simulink model "controlador_PID"  (R2018a)
settings: Solver=VariableStepAuto  StartTime=0.0  StopTime=10.0  RelTol=1e-3
values from neighbouring files (symbols this model uses):
  b_a = J_eq * n * w_pos    (= 0.0113019895361)    [proyecto_global_integrador.m]
  k_sa = J_eq * n * w_pos^2    (= 9.04159162887)    [proyecto_global_integrador.m]
  k_sia = J_eq * w_pos^3    (= 2893.30932124)    [proyecto_global_integrador.m]
settings Model: Creator=gabrielq  LastModifiedBy=gabrielq

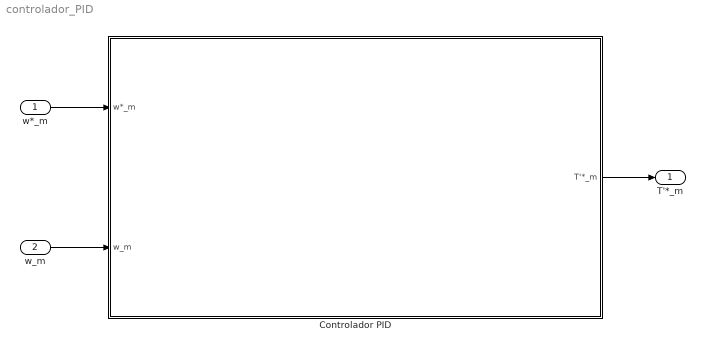
== system controlador_PID ==
  w*_m : Inport
  w_m : Inport  Port=2
  Controlador PID : Subsystem
  T'*_m : Outport
  wires:
  w*_m/1 -> Controlador PID/1(w*_m)
  w_m/1 -> Controlador PID/2(w_m)
  Controlador PID/1(T'*_m) -> T'*_m/1

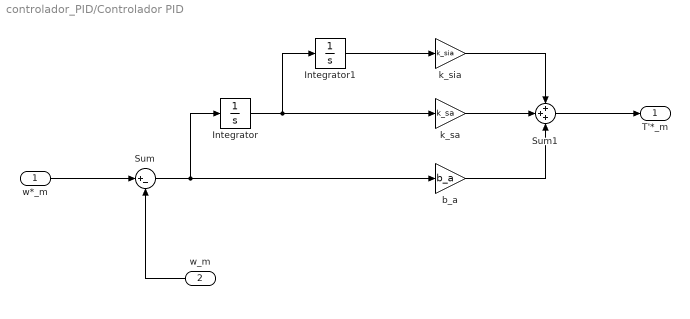
== system controlador_PID/Controlador PID ==
  w*_m : Inport
  w_m : Inport  Port=2
  Integrator : Integrator
  Integrator1 : Integrator
  Sum : Sum  Inputs=|+-
  Sum1 : Sum  Inputs=+++
  b_a : Gain  Gain=b_a
  k_sa : Gain  Gain=k_sa
  k_sia : Gain  Gain=k_sia
  T'*_m : Outport
  wires:
  w_m/1 -> Sum/2
  b_a/1 -> Sum1/3
  Integrator1/1 -> k_sia/1
  k_sia/1 -> Sum1/1
  w*_m/1 -> Sum/1
  Sum/1 -> Integrator/1, b_a/1
  k_sa/1 -> Sum1/2
  Sum1/1 -> T'*_m/1
  Integrator/1 -> Integrator1/1, k_sa/1
